simulink library "INT_InjVlv_CalcET"  (R2016b)
settings: Solver=VariableStepAuto  StartTime=0.0  StopTime=10.0  RelTol=1e-3
settings Model: Creator=mayongchao  LastModifiedBy=mayongchao

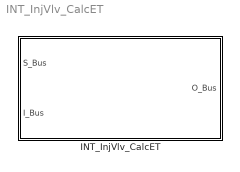
== system INT_InjVlv_CalcET ==
  INT_InjVlv_CalcET : Subsystem

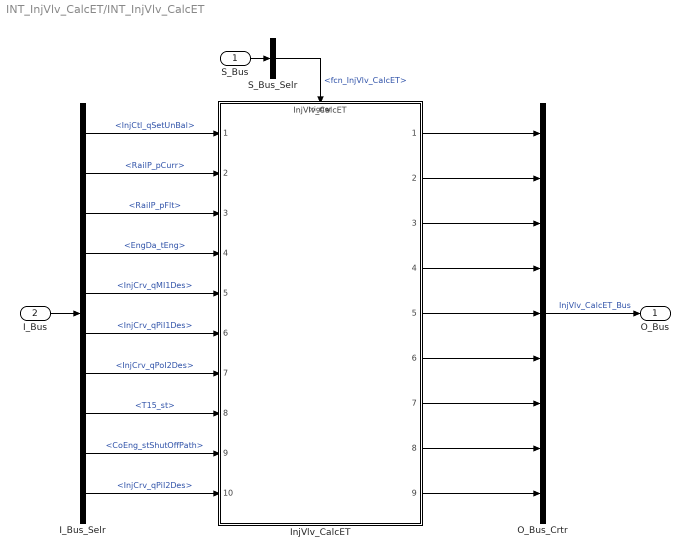
== system INT_InjVlv_CalcET/INT_InjVlv_CalcET ==
  S_Bus : Inport
  I_Bus : Inport  Port=2
  I_Bus_Selr : BusSelector  OutputSignals=InjCtl_qSetUnBal,RailP_pCurr,RailP_pFlt,EngDa_tEng,InjCrv_qMI1Des,InjCrv_qPiI1Des,InjCrv_qPoI2Des,T15_st,CoEng_stShutOffPath,InjCrv_qPiI2Des
  InjVlv_CalcET : ModelReference  ModelNameDialog=InjVlv_CalcET  SimulationMode=Normal  ModelReferenceVersion=1.43  TriggerPortName=function  TriggerPortTriggerType=function-call  TriggerPortStatesWhenEnabling=held
  O_Bus_Crtr : BusCreator  Inputs=9
  S_Bus_Selr : BusSelector  OutputSignals=fcn_InjVlv_CalcET
  O_Bus : Outport
  wires:
  S_Bus_Selr/1 -> InjVlv_CalcET/Trigger  "<fcn_InjVlv_CalcET>"
  S_Bus/1 -> S_Bus_Selr/1
  I_Bus/1 -> I_Bus_Selr/1
  I_Bus_Selr/1 -> InjVlv_CalcET/1  "<InjCtl_qSetUnBal>"
  I_Bus_Selr/2 -> InjVlv_CalcET/2  "<RailP_pCurr>"
  I_Bus_Selr/3 -> InjVlv_CalcET/3  "<RailP_pFlt>"
  I_Bus_Selr/4 -> InjVlv_CalcET/4  "<EngDa_tEng>"
  I_Bus_Selr/5 -> InjVlv_CalcET/5  "<InjCrv_qMI1Des>"
  I_Bus_Selr/6 -> InjVlv_CalcET/6  "<InjCrv_qPiI1Des>"
  I_Bus_Selr/7 -> InjVlv_CalcET/7  "<InjCrv_qPoI2Des>"
  I_Bus_Selr/8 -> InjVlv_CalcET/8  "<T15_st>"
  I_Bus_Selr/9 -> InjVlv_CalcET/9  "<CoEng_stShutOffPath>"
  I_Bus_Selr/10 -> InjVlv_CalcET/10  "<InjCrv_qPiI2Des>"
  O_Bus_Crtr/1 -> O_Bus/1  "InjVlv_CalcET_Bus"
  InjVlv_CalcET/1 -> O_Bus_Crtr/1
  InjVlv_CalcET/2 -> O_Bus_Crtr/2
  InjVlv_CalcET/3 -> O_Bus_Crtr/3
  InjVlv_CalcET/4 -> O_Bus_Crtr/4
  InjVlv_CalcET/5 -> O_Bus_Crtr/5
  InjVlv_CalcET/6 -> O_Bus_Crtr/6
  InjVlv_CalcET/7 -> O_Bus_Crtr/7
  InjVlv_CalcET/8 -> O_Bus_Crtr/8
  InjVlv_CalcET/9 -> O_Bus_Crtr/9
